simulink model "untitled"  (Simulink 8.1)
settings: Solver=ode45  StartTime=0.0  StopTime=1  RelTol=1e-3
settings Model: Creator=DELL  LastModifiedBy=DELL
settings DataIOCC: SignalLoggingSaveFormat=Dataset
settings OptimizationCC: ExpressionDepthLimit=128
settings DebuggingCC: FcnCallInpInsideContextMsg=EnableAllAsError
settings GRTTargetCC: CombineOutputUpdateFcns=on  GRTInterface=off

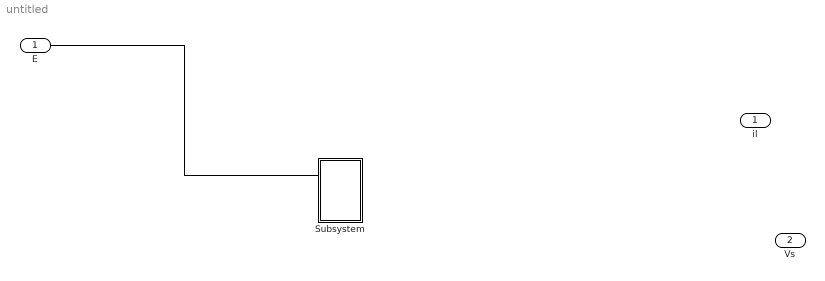
== system untitled ==
  E : Inport
  Subsystem : Subsystem
  il : Outport
  Vs : Outport  Port=2
  wires:
  E/1 -> ?
  ? -> il/1
  ? -> Vs/1

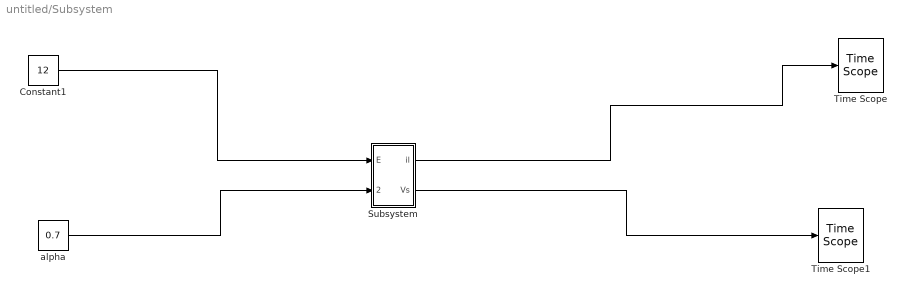
== system untitled/Subsystem ==
  Constant1 : Constant  Value=12
  Subsystem : Subsystem
  Time Scope : TimeScope  DefaultConfigurationName=spbscopes.TimeScopeBlockCfg
      settings: CopyFcn=scopeextensions.ScopeBlock.callback(gcbh, 'onBlockCopy', gcbh);  DeleteFcn=scopeextensions.ScopeBlock.callback(gcbh, 'onBlockDelete');  PreSaveFcn=scopeextensions.ScopeBlock.callback(gcbh, 'onModelSave');  NameChangeFcn=scopeextensions.ScopeBlock.callback(gcbh, 'onBlockRename');  CloseFcn=scopeextensions.ScopeBlock.callback(gcbh, 'onBlockClose');  PreDeleteFcn=scopeextensions.ScopeBlock.callback(gcbh, 'onBlockPreDelete');
  Time Scope1 : TimeScope  DefaultConfigurationName=spbscopes.TimeScopeBlockCfg
      settings: CopyFcn=scopeextensions.ScopeBlock.callback(gcbh, 'onBlockCopy', gcbh);  DeleteFcn=scopeextensions.ScopeBlock.callback(gcbh, 'onBlockDelete');  PreSaveFcn=scopeextensions.ScopeBlock.callback(gcbh, 'onModelSave');  NameChangeFcn=scopeextensions.ScopeBlock.callback(gcbh, 'onBlockRename');  CloseFcn=scopeextensions.ScopeBlock.callback(gcbh, 'onBlockClose');  PreDeleteFcn=scopeextensions.ScopeBlock.callback(gcbh, 'onBlockPreDelete');
  "alpha " : Constant  Value=0.7
  wires:
  Subsystem/1(il) -> Time Scope/1
  Subsystem/2(Vs) -> Time Scope1/1
  Constant1/1 -> Subsystem/1(E)
  "alpha "/1 -> Subsystem/2("alpha ")

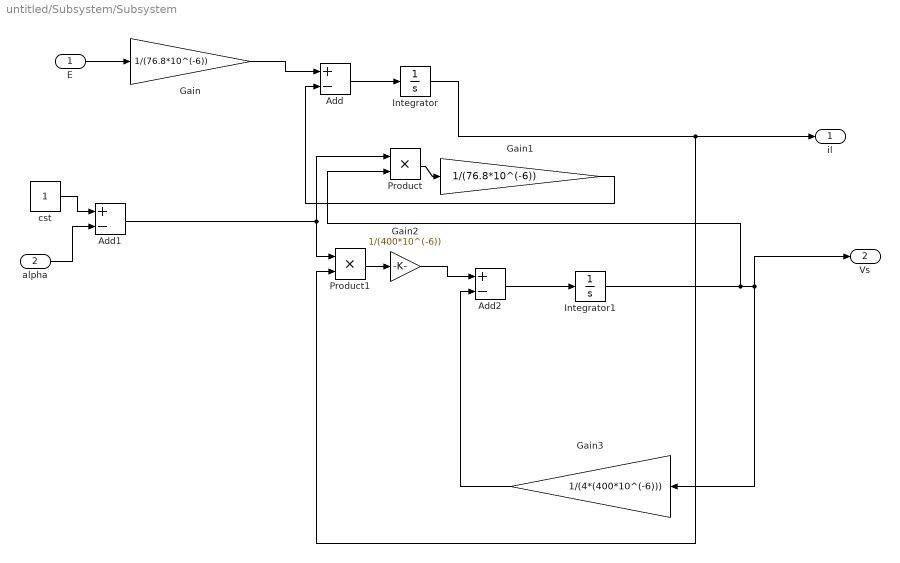
== system untitled/Subsystem/Subsystem ==
  E : Inport
  "alpha " : Inport  Port=2
  Add : Sum  Inputs=+-
  Add1 : Sum  Inputs=+-
  Add2 : Sum  Inputs=+-
  Gain : Gain  Gain=1/(76.8*10^(-6))
  Gain1 : Gain  Gain=1/(76.8*10^(-6))
  Gain2 : Gain  Gain=1/(400*10^(-6))
  Gain3 : Gain  Gain=1/(4*(400*10^(-6)))
  Integrator : Integrator
  Integrator1 : Integrator
  Product : Product
  Product1 : Product
  "cst " : Constant
  il : Outport
  Vs : Outport  Port=2
  wires:
  Add2/1 -> Integrator1/1
  Gain2/1 -> Add2/1
  Gain3/1 -> Add2/2
  E/1 -> Gain/1
  Add1/1 -> Product/1, Product1/1
  Add/1 -> Integrator/1
  Gain1/1 -> Add/2
  "cst "/1 -> Add1/1
  Gain/1 -> Add/1
  Product/1 -> Gain1/1
  Integrator/1 -> il/1, Product1/2
  Product1/1 -> Gain2/1
  Integrator1/1 -> Product/2, Vs/1, Gain3/1
  "alpha "/1 -> Add1/2
